simulink model "quad_integrator_subsys_2delays"  (Simulink 7.3)
settings: Solver=ode45  StartTime=0.0  StopTime=10*30  FixedStep=.0001  MaxStep=.02  RelTol=1e-3
InitFcn:
  | Ts=0.02;
settings Model: Creator=jporter  LastModifiedBy=jporter
settings OptimizationCC: InitFltsAndDblsToZero=on

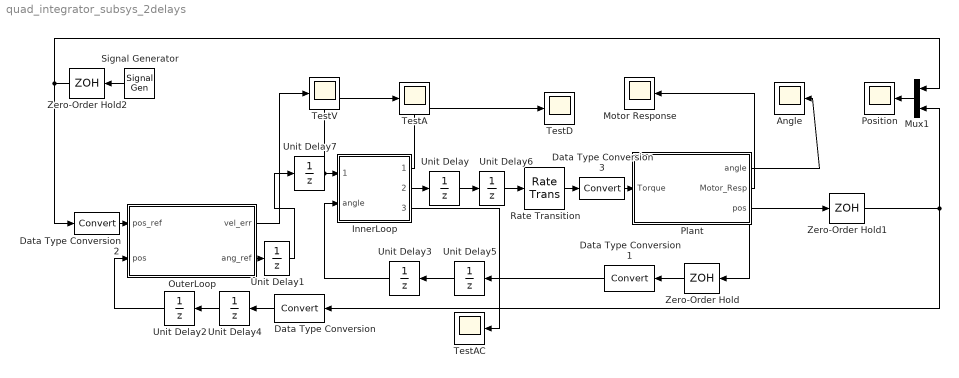
== system quad_integrator_subsys_2delays ==
  Angle : Scope
  Data Type Conversion{,1..3} (4 alike) : DataTypeConversion  OutDataType=sfix(16)  OutScaling=2^0
  InnerLoop : Subsystem
  Motor Response : Scope
      settings: TimeRange=500  YMin=-40  YMax=40  SaveName=ScopeData2
  Mux1 : Mux  Inputs=2
  OuterLoop : Subsystem
  Plant : Subsystem
  Position : Scope
      settings: YMin=-20  YMax=20  SaveName=Pos2Delay
  Rate Transition : RateTransition
  Signal Generator : SignalGenerator  WaveForm=square  Frequency=1/30
  TestA : Scope
      settings: YMin=-75  YMax=100  SaveName=ScopeData4
  TestAC : Scope
      settings: SaveName=ScopeData6
  TestD : Scope
      settings: SaveName=ScopeData3
  TestV : Scope
      settings: SaveName=ScopeData5
  Unit Delay{,1..7} (8 alike) : UnitDelay  SampleTime=Ts
  Zero-Order Hold : ZeroOrderHold  SampleTime=Ts
  Zero-Order Hold1 : ZeroOrderHold  SampleTime=Ts
  Zero-Order Hold2 : ZeroOrderHold  SampleTime=Ts
  wires:
  InnerLoop/2(Torque) -> Unit Delay/1
  Plant/3(pos) -> Zero-Order Hold1/1
  Mux1/1 -> Position/1
  Signal Generator/1 -> Zero-Order Hold2/1
  InnerLoop/1(ang_err) -> TestD/1
  InnerLoop/3(ang_vel) -> TestAC/1
  Plant/1(angle) -> Angle/1, Zero-Order Hold/1
  Plant/2(Motor_Resp) -> Motor Response/1
  OuterLoop/2(ang_ref) -> Unit Delay1/1
  OuterLoop/1(vel_err) -> TestV/1
  Data Type Conversion/1 -> Unit Delay4/1
  Data Type Conversion1/1 -> Unit Delay5/1
  Data Type Conversion2/1 -> OuterLoop/1(pos_ref)
  Data Type Conversion3/1 -> Plant/1(Torque)
  Zero-Order Hold/1 -> Data Type Conversion1/1
  Zero-Order Hold2/1 -> Mux1/1, Data Type Conversion2/1
  Rate Transition/1 -> Data Type Conversion3/1
  Zero-Order Hold1/1 -> Mux1/2, Data Type Conversion/1
  Unit Delay/1 -> Unit Delay6/1
  Unit Delay2/1 -> OuterLoop/2(pos)
  Unit Delay3/1 -> InnerLoop/2(angle)
  Unit Delay4/1 -> Unit Delay2/1
  Unit Delay5/1 -> Unit Delay3/1
  Unit Delay6/1 -> Rate Transition/1
  Unit Delay1/1 -> Unit Delay7/1
  Unit Delay7/1 -> InnerLoop/1(ang_ref), TestA/1

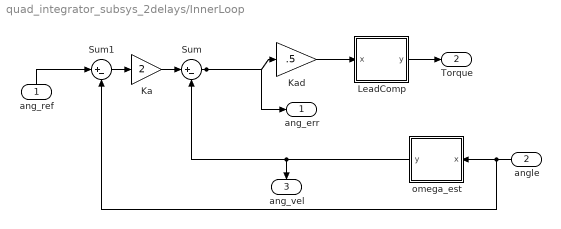
== system quad_integrator_subsys_2delays/InnerLoop ==
  ang_ref : Inport  DataType=single  OutDataTypeStr=single
  angle : Inport  Port=2  DataType=single  OutDataTypeStr=single
  Ka : Gain  Gain=2  ParameterDataTypeMode=single  ParameterDataType=sfix(16)  ParameterScaling=2^0  ParamDataTypeStr=single  OutDataType=sfix(16)  OutScaling=2^0
  Kad : Gain  Gain=.5  ParameterDataTypeMode=single  ParameterDataType=sfix(16)  ParameterScaling=2^0  ParamDataTypeStr=single  OutDataType=sfix(16)  OutScaling=2^0
  LeadComp : Subsystem
  Sum : Sum  Inputs=|+-  OutDataType=sfix(16)  OutScaling=2^0
  Sum1 : Sum  Inputs=|+-  OutDataType=sfix(16)  OutScaling=2^0
  omega_est : Subsystem
  ang_err : Outport
  Torque : Outport  Port=2  DataType=single  OutDataTypeStr=single
  ang_vel : Outport  Port=3
  wires:
  Sum1/1 -> Ka/1
  Ka/1 -> Sum/1
  Sum/1 -> Kad/1, ang_err/1
  Kad/1 -> LeadComp/1(x)
  omega_est/1(y) -> Sum/2, ang_vel/1
  angle/1 -> Sum1/2, omega_est/1(x)
  LeadComp/1(y) -> Torque/1
  ang_ref/1 -> Sum1/1

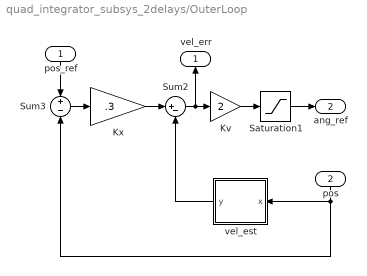
== system quad_integrator_subsys_2delays/OuterLoop ==
  pos_ref : Inport  DataType=single  OutDataTypeStr=single
  pos : Inport  Port=2  DataType=single  OutDataTypeStr=single
  Kv : Gain  Gain=2  ParameterDataTypeMode=single  ParameterDataType=sfix(16)  ParameterScaling=2^0  ParamDataTypeStr=single  OutDataType=sfix(16)  OutScaling=2^0
  Kx : Gain  Gain=.3  ParameterDataTypeMode=single  ParameterDataType=sfix(16)  ParameterScaling=2^0  ParamDataTypeStr=single  OutDataType=sfix(16)  OutScaling=2^0
  Saturation1 : Saturate  UpperLimit=pi/4  LowerLimit=-pi/4  OutDataType=sfix(16)  OutScaling=2^0
  Sum2 : Sum  Inputs=|+-  OutDataType=sfix(16)  OutScaling=2^0
  Sum3 : Sum  Inputs=+|-  OutDataType=sfix(16)  OutScaling=2^0
  vel_est : Subsystem
  vel_err : Outport
  ang_ref : Outport  Port=2  DataType=single  OutDataTypeStr=single
  wires:
  Kx/1 -> Sum2/1
  Sum2/1 -> Kv/1, vel_err/1
  Kv/1 -> Saturation1/1
  vel_est/1(y) -> Sum2/2
  Sum3/1 -> Kx/1
  pos_ref/1 -> Sum3/1
  Saturation1/1 -> ang_ref/1
  pos/1 -> Sum3/2, vel_est/1(x)

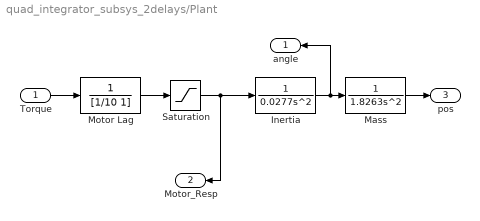
== system quad_integrator_subsys_2delays/Plant ==
  Torque : Inport
  Inertia : TransferFcn  Denominator=[0.0277 0 0]
  Mass : TransferFcn  Denominator=[1.8263 0 0]
  Motor Lag : TransferFcn  Denominator=[1/10 1]
  Saturation : Saturate  UpperLimit=40  LowerLimit=-40  OutDataType=sfix(16)  OutScaling=2^0
  angle : Outport
  Motor_Resp : Outport  Port=2
  pos : Outport  Port=3
  wires:
  Motor Lag/1 -> Saturation/1
  Saturation/1 -> Inertia/1, Motor_Resp/1
  Inertia/1 -> Mass/1, angle/1
  Mass/1 -> pos/1
  Torque/1 -> Motor Lag/1

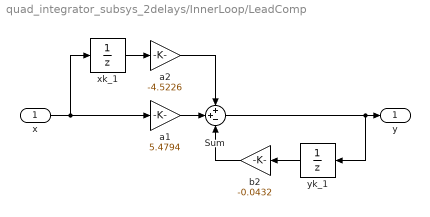
== system quad_integrator_subsys_2delays/InnerLoop/LeadComp ==
  x : Inport  OutDataType=sfix(16)  OutScaling=2^0
  Sum : Sum  Inputs=++-  OutDataType=sfix(16)  OutScaling=2^0
  a1 : Gain  Gain=5.4794  ParameterDataTypeMode=single  ParameterDataType=sfix(16)  ParameterScaling=2^0  ParamDataTypeStr=single  OutDataType=sfix(16)  OutScaling=2^0
  a2 : Gain  Gain=-4.5226  ParameterDataTypeMode=single  ParameterDataType=sfix(16)  ParameterScaling=2^0  ParamDataTypeStr=single  OutDataType=sfix(16)  OutScaling=2^0
  b2 : Gain  Gain=-0.0432  ParameterDataTypeMode=single  ParameterDataType=sfix(16)  ParameterScaling=2^0  ParamDataTypeStr=single  OutDataType=sfix(16)  OutScaling=2^0
  xk_1 : UnitDelay  SampleTime=Ts
  yk_1 : UnitDelay  SampleTime=Ts
  y : Outport  OutDataType=sfix(16)  OutScaling=2^0
  wires:
  b2/1 -> Sum/3
  yk_1/1 -> b2/1
  Sum/1 -> y/1, yk_1/1
  a1/1 -> Sum/2
  a2/1 -> Sum/1
  xk_1/1 -> a2/1
  x/1 -> xk_1/1, a1/1

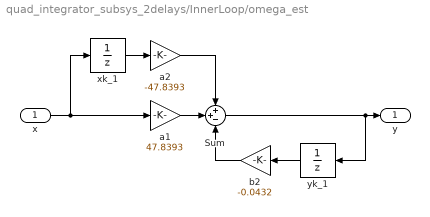
== system quad_integrator_subsys_2delays/InnerLoop/omega_est ==
  x : Inport  OutDataType=sfix(16)  OutScaling=2^0
  Sum : Sum  Inputs=++-  OutDataType=sfix(16)  OutScaling=2^0
  a1 : Gain  Gain=47.8393  ParameterDataTypeMode=single  ParameterDataType=sfix(16)  ParameterScaling=2^0  ParamDataTypeStr=single  OutDataType=sfix(16)  OutScaling=2^0
  a2 : Gain  Gain=-47.8393  ParameterDataTypeMode=single  ParameterDataType=sfix(16)  ParameterScaling=2^0  ParamDataTypeStr=single  OutDataType=sfix(16)  OutScaling=2^0
  b2 : Gain  Gain=-0.0432  ParameterDataTypeMode=single  ParameterDataType=sfix(16)  ParameterScaling=2^0  ParamDataTypeStr=single  OutDataType=sfix(16)  OutScaling=2^0
  xk_1 : UnitDelay  SampleTime=Ts
  yk_1 : UnitDelay  SampleTime=Ts
  y : Outport  OutDataType=sfix(16)  OutScaling=2^0
  wires:
  b2/1 -> Sum/3
  yk_1/1 -> b2/1
  Sum/1 -> y/1, yk_1/1
  a1/1 -> Sum/2
  a2/1 -> Sum/1
  xk_1/1 -> a2/1
  x/1 -> xk_1/1, a1/1

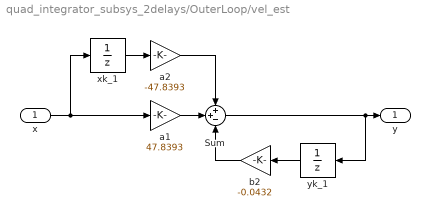
== system quad_integrator_subsys_2delays/OuterLoop/vel_est ==
  x : Inport  OutDataType=sfix(16)  OutScaling=2^0
  Sum : Sum  Inputs=++-  OutDataType=sfix(16)  OutScaling=2^0
  a1 : Gain  Gain=47.8393  ParameterDataTypeMode=single  ParameterDataType=sfix(16)  ParameterScaling=2^0  ParamDataTypeStr=single  OutDataType=sfix(16)  OutScaling=2^0
  a2 : Gain  Gain=-47.8393  ParameterDataTypeMode=single  ParameterDataType=sfix(16)  ParameterScaling=2^0  ParamDataTypeStr=single  OutDataType=sfix(16)  OutScaling=2^0
  b2 : Gain  Gain=-0.0432  ParameterDataTypeMode=single  ParameterDataType=sfix(16)  ParameterScaling=2^0  ParamDataTypeStr=single  OutDataType=sfix(16)  OutScaling=2^0
  xk_1 : UnitDelay  SampleTime=Ts
  yk_1 : UnitDelay  SampleTime=Ts
  y : Outport  OutDataType=sfix(16)  OutScaling=2^0
  wires:
  x/1 -> a1/1, xk_1/1
  xk_1/1 -> a2/1
  a2/1 -> Sum/1
  a1/1 -> Sum/2
  Sum/1 -> yk_1/1, y/1
  yk_1/1 -> b2/1
  b2/1 -> Sum/3
